simulink model "pos_servo_control_simu"  (R2020b)
settings: Solver=VariableStepAuto  StartTime=0.0  StopTime=tfinal  RelTol=1e-3
values from neighbouring files (symbols this model uses):
  A = [0,1;0,-1/T]    [exp_pos_state_control.m]    (also in pos_state_control.m; pos_state_control1.m)
  B = [0;K/T]    [exp_pos_state_control.m]    (also in pos_state_control.m; pos_state_control1.m)
  C = [1,0]    [exp_pos_state_control.m]    (also in pos_state_control.m; pos_state_control1.m)
  F = F_bar(1:2)    [exp_pos_state_control.m]    (also in pos_state_control.m)
  Ki = -F_bar(3)    [exp_pos_state_control.m]    (also in pos_state_control.m)
  r = 60    [exp_pos_state_control.m]    (also in pos_state_control.m; pos_state_control1.m)
  r_cyc = 8    [exp_pos_state_control.m]    (also in pos_state_control.m; pos_state_control1.m)
  x0 = [theta0;omega0]    [exp_pos_state_control.m]    (also in pos_state_control.m; pos_state_control1.m)
libraries: arduino_io_lib x2
settings Model: Creator=kei55  LastModifiedBy=kei55

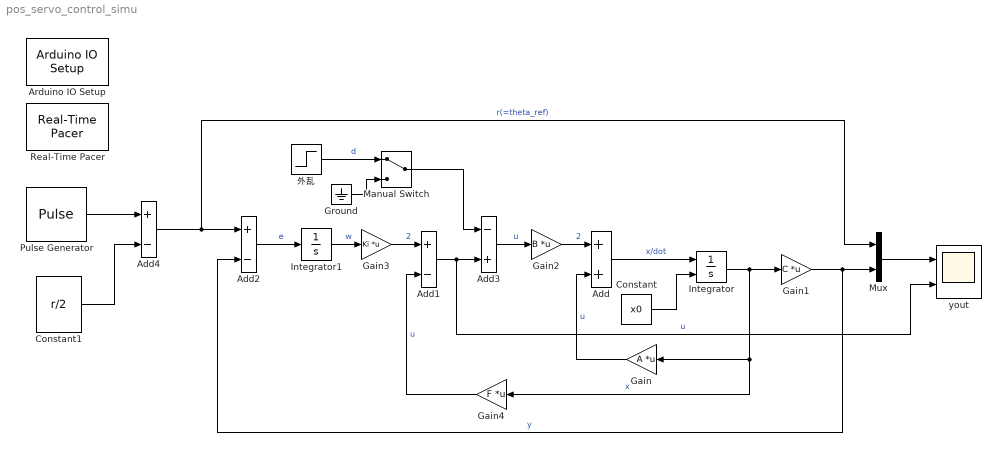
== system pos_servo_control_simu ==
  Add : Sum
  Add1 : Sum  Inputs=+-
  Add2 : Sum  Inputs=+-
  Add3 : Sum  Inputs=-+
  Add4 : Sum  Inputs=+-
  Arduino IO Setup : arduino_io_lib/Arduino IO Setup  Priority=3  arduinoVar=Temporary arduino variable: Arduino1  workspaceVarName=a  comPort=COM3
  Constant : Constant  Value=x0  VectorParams1D=off
  Constant1 : Constant  Value=r/2
  Gain : Gain  Gain=A  Multiplication=Matrix(K*u)
  Gain1 : Gain  Gain=C  Multiplication=Matrix(K*u)
  Gain2 : Gain  Gain=B  Multiplication=Matrix(K*u)
  Gain3 : Gain  Gain=Ki  Multiplication=Matrix(K*u)
  Gain4 : Gain  Gain=F  Multiplication=Matrix(K*u)
  Ground : Ground
  Integrator : Integrator  InitialConditionSource=external
  Integrator1 : Integrator
  Manual Switch : ManualSwitch
  Mux : Mux  Inputs=2
  Pulse Generator : DiscretePulseGenerator  PulseType=Time based  Amplitude=r  Period=r_cyc  PulseWidth=50  SampleTime=1/50
  Real-Time Pacer : arduino_io_lib/Real-Time Pacer  simTimePerRealTime=1
  yout : Scope  NumInputPorts=2
  外乱 : Step  SampleTime=0
  wires:
  Add/1 -> Integrator/1  "x/dot"
  Integrator/1 -> Gain1/1, Gain4/1, Gain/1  "x"
  Gain2/1 -> Add/1  "2"
  Gain/1 -> Add/2  "u"
  Gain1/1 -> Mux/2, Add2/2  "y"
  Constant/1 -> Integrator/2
  Gain3/1 -> Add1/1  "2"
  Add4/1 -> Add2/1, Mux/1  "r(=theta_ref)"
  Add2/1 -> Integrator1/1  "e"
  Gain4/1 -> Add1/2  "u"
  Constant1/1 -> Add4/2
  Pulse Generator/1 -> Add4/1
  Integrator1/1 -> Gain3/1  "w"
  Add1/1 -> yout/2, Add3/2  "u"
  Add3/1 -> Gain2/1  "u"
  Manual Switch/1 -> Add3/1
  外乱/1 -> Manual Switch/1  "d"
  Ground/1 -> Manual Switch/2
  Mux/1 -> yout/1
